simulink model "VerificaLQR"  (R2025b)
settings: Solver=VariableStepAuto  StartTime=0.0  StopTime=10.0  RelTol=1e-3
undefined symbols (not defined in the file): A, B, C, C_sel, D, K_LQR_i, K_LQR_x, q1_ref_LQR
settings Model: Creator=salvo  LastModifiedBy=salvo

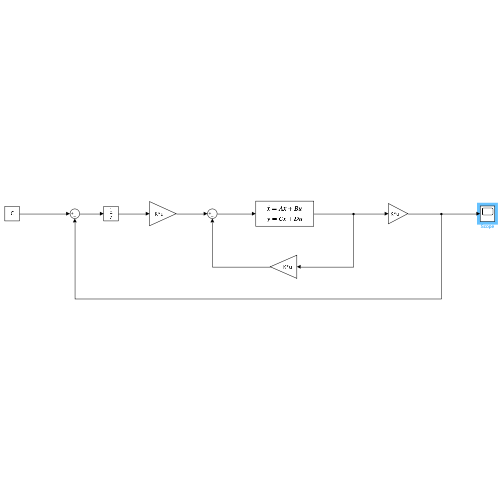
[thumbnail: Simulink's stored preview of the top-level diagram]
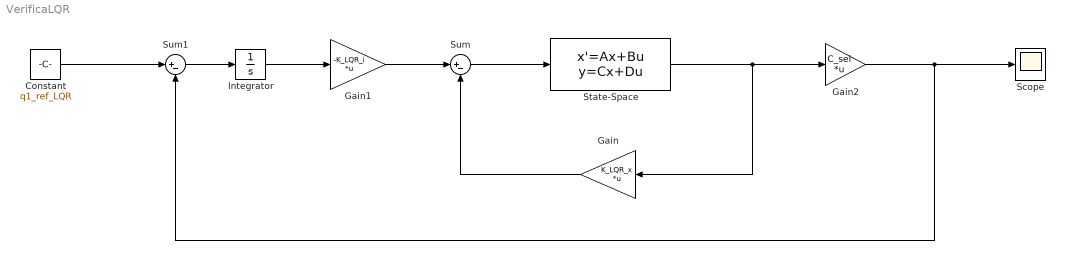
== system VerificaLQR ==
  Constant : Constant  Value=q1_ref_LQR
  Gain : Gain  Gain=K_LQR_x  Multiplication=Matrix(K*u)
  Gain1 : Gain  Gain=-K_LQR_i  Multiplication=Matrix(K*u)
  Gain2 : Gain  Gain=C_sel  Multiplication=Matrix(K*u)
  Integrator : Integrator
  Scope : Scope
      settings: ActiveDisplayYMinimum=-2.0217430786591413  ActiveDisplayYMaximum=2.6058882749871763
  State-Space : StateSpace  A=A  B=B  C=C  D=D  InitialCondition=0
  Sum : Sum  Inputs=|+-
  Sum1 : Sum  Inputs=|+-
  wires:
  State-Space/1 -> Gain/1, Gain2/1
  Gain/1 -> Sum/2
  Sum/1 -> State-Space/1
  Gain1/1 -> Sum/1
  Integrator/1 -> Gain1/1
  Sum1/1 -> Integrator/1
  Constant/1 -> Sum1/1
  Gain2/1 -> Sum1/2, Scope/1
